simulink model "three_phase_inverter"  (R2025a)
settings: Solver=VariableStepAuto  StartTime=0.0  StopTime=1  FixedStep=step_time
undefined symbols (not defined in the file): fsw, Ls, Rs, Vdc
libraries: spsMosfetLib x6, spsVoltageMeasurementLib x6, spsCurrentMeasurementLib x3, spsDCVoltageSourceLib x2, ee_lib x2, nesl_utility x1, spsThreePhaseSeriesRLCBranchLib x1, fl_lib x1, spspowerguiLib x1
settings Model: Creator=moon  LastModifiedBy=moon

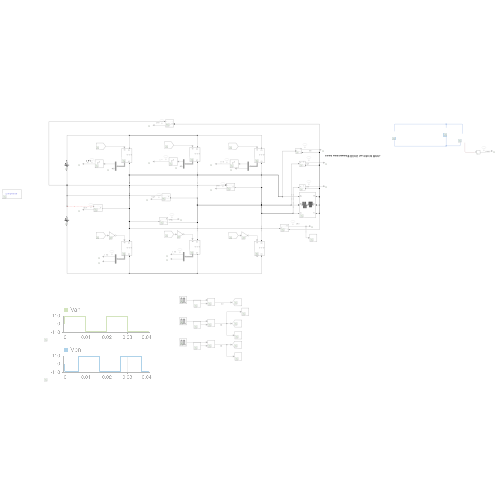
[thumbnail: Simulink's stored preview of the top-level diagram]
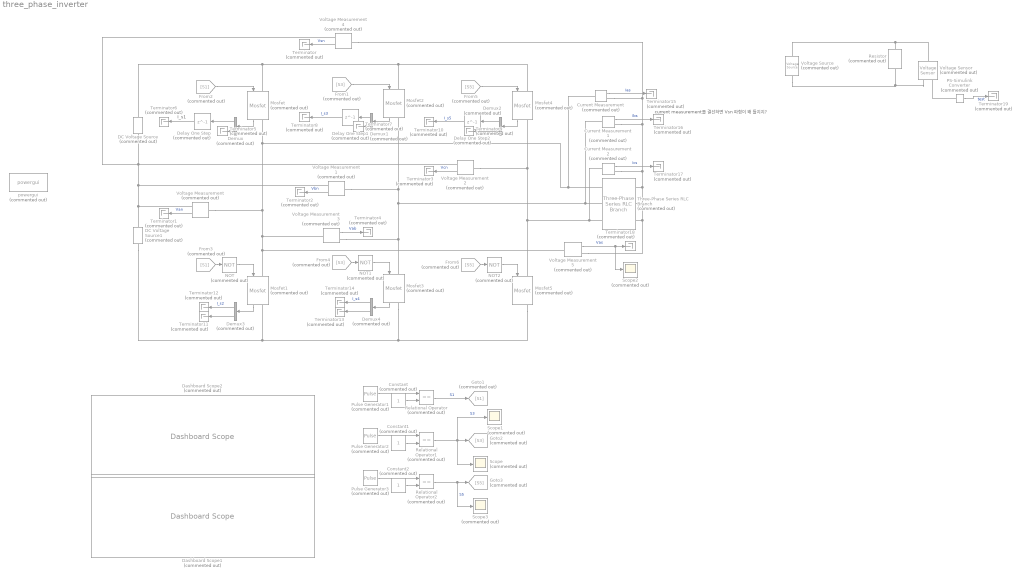
== system three_phase_inverter ==
  note: I_s1
  note: current measurement를 결선하면 Vsn 파형이 왜 틀지지?
  Constant : Constant  Commented=on
  Constant1 : Constant  Commented=on
  Constant2 : Constant  Commented=on
  Current Measurement : spsCurrentMeasurementLib/Current Measurement  Commented=on  PhasorSimulation=off  OutputType=Complex  PSBequivalent=0
  Current Measurement1 : spsCurrentMeasurementLib/Current Measurement  Commented=on  PhasorSimulation=off  OutputType=Complex  PSBequivalent=0
  Current Measurement2 : spsCurrentMeasurementLib/Current Measurement  Commented=on  PhasorSimulation=off  OutputType=Complex  PSBequivalent=0
  DC Voltage Source : spsDCVoltageSourceLib/DC Voltage Source  Commented=on  Amplitude=Vdc  Measurements=None
  DC Voltage Source1 : spsDCVoltageSourceLib/DC Voltage Source  Commented=on  Amplitude=Vdc  Measurements=None
  Dashboard Scope1 : DashboardScope  Commented=on  FontColor=[0.0, 0.0, 0.0]
  Dashboard Scope2 : DashboardScope  Commented=on  FontColor=[0.0, 0.0, 0.0]
  Delay One Step : Delay  Commented=on  DelayLength=1
  Delay One Step1 : Delay  Commented=on  DelayLength=1
  Delay One Step2 : Delay  Commented=on  DelayLength=1
  Demux{,1..4} (5 alike) : Demux  Commented=on  Outputs=2
  From1 : From  Commented=on  GotoTag=S3
  From2 : From  Commented=on  GotoTag=S1
  From3 : From  Commented=on  GotoTag=S1
  From4 : From  Commented=on  GotoTag=S3
  From5 : From  Commented=on  GotoTag=S5
  From6 : From  Commented=on  GotoTag=S5
  Goto1 : Goto  Commented=on  GotoTag=S1
  Goto2 : Goto  Commented=on  GotoTag=S3
  Goto3 : Goto  Commented=on  GotoTag=S5
  Mosfet{,1..5} (6 alike) : spsMosfetLib/Mosfet  Commented=on  Ron=R_FET  Lon=0  Rd=R_Diode  Vfd=0  IC=0  Rs=1e5  Cs=inf  Measurements=on
  NOT : Logic  Commented=on  Operator=NOT  IconShape=distinctive  AllPortsSameDT=off  OutDataTypeStr=boolean
  NOT1 : Logic  Commented=on  Operator=NOT  IconShape=distinctive  AllPortsSameDT=off  OutDataTypeStr=boolean
  NOT2 : Logic  Commented=on  Operator=NOT  IconShape=distinctive  AllPortsSameDT=off  OutDataTypeStr=boolean
  PS-Simulink Converter : nesl_utility/PS-Simulink Converter  Commented=on  PhysicalDomain=network_engine_domain  SubClassName=ps_output  LeftPortType=input  RightPortType=output  PseudoPeriodic=off  Frequencies=[]  VectorFormat=inherit  Unit=inherit  AffineConversion=off
  Pulse Generator1 : DiscretePulseGenerator  Commented=on  PulseType=Time based  Period=1/fsw  PulseWidth=50
  Pulse Generator2 : DiscretePulseGenerator  Commented=on  PulseType=Time based  Period=1/fsw  PulseWidth=50  PhaseDelay=1/fsw/3
  Pulse Generator3 : DiscretePulseGenerator  Commented=on  PulseType=Time based  Period=1/fsw  PulseWidth=50  PhaseDelay=-1/fsw/3
  Relational Operator : RelationalOperator  Commented=on  Operator===  OutDataTypeStr=boolean  RndMeth=Simplest  InputSameDT=off
  Relational Operator1 : RelationalOperator  Commented=on  Operator===  OutDataTypeStr=boolean  RndMeth=Simplest  InputSameDT=off
  Relational Operator2 : RelationalOperator  Commented=on  Operator===  OutDataTypeStr=boolean  RndMeth=Simplest  InputSameDT=off
  Resistor : ee_lib/Passive/Resistor  Commented=on  R=1 Ohm  enable_R_tol=ee.enum.toleranceApplication.none  R_tol=5  tol_distribution=ee.enum.toleranceDistribution.uniform  nSigma=4  enable_operating_limits=ee.enum.enable.no  operating_limit_action=ee.enum.passive.reportOpLim.warn  power_rating=1 W  max_working_voltage=100 V  noise_mode=ee.enum.sources.noise.Disabled  Tdevice=25 degC  sample_time=1e-3 s  repeatability=ee.enum.ic.repeatability.notRepeatable  user_seed=0  auto_seed=2715962282  power_derating_T1=70 degC  power_derating_T2=155 degC  operating_temperature_range_vec=[-50, 150] degC  alpha=3.93e-3 1/K  Tmeas=25 degC  thermal_mass=100 J/K  temperature_specify=off  temperature_priority=High  temperature=298.15 K  temperature_nominal_specify=off  temperature_nominal_value=1  temperature_nominal_unit=K
  Scope{,1..3} (4 alike) : Scope  Commented=on
      Scope settings: ActiveDisplayYMinimum=-0.12499999999999997  ActiveDisplayYMaximum=1.125
      Scope1 settings: ActiveDisplayYMinimum=-0.12499999999999997  ActiveDisplayYMaximum=1.125
      Scope2 settings: ActiveDisplayYMinimum=-166.66666666666666  ActiveDisplayYMaximum=166.66666666666663  DataLoggingVariableName=ScopeData2
      Scope3 settings: ActiveDisplayYMinimum=-1  ActiveDisplayYMaximum=1  DataLoggingVariableName=ScopeData3
  Terminator{,1..19} (20 alike) : Terminator  Commented=on
  Three-Phase Series RLC Branch : spsThreePhaseSeriesRLCBranchLib/Three-Phase Series RLC Branch  Commented=on  LConnTagsString=A|B|C  RConnTagsString=A|B|C  BranchType=RL  Resistance=Rs  Inductance=Ls  Capacitance=1e-6  Measurements=Branch voltages and currents
  Voltage Measurement : spsVoltageMeasurementLib/Voltage Measurement  Commented=on  PhasorSimulation=off  OutputType=Complex  PSBequivalent=0
      link override -: Side=Right
  Voltage Measurement1 : spsVoltageMeasurementLib/Voltage Measurement  Commented=on  PhasorSimulation=off  OutputType=Complex  PSBequivalent=0
      link override -: Side=Right
  Voltage Measurement2 : spsVoltageMeasurementLib/Voltage Measurement  Commented=on  PhasorSimulation=off  OutputType=Complex  PSBequivalent=0
      link override -: Side=Right
  Voltage Measurement3 : spsVoltageMeasurementLib/Voltage Measurement  Commented=on  PhasorSimulation=off  OutputType=Complex  PSBequivalent=0
      link override -: Side=Right
  Voltage Measurement4 : spsVoltageMeasurementLib/Voltage Measurement  Commented=on  PhasorSimulation=off  OutputType=Complex  PSBequivalent=0
      link override -: Side=Right
  Voltage Measurement5 : spsVoltageMeasurementLib/Voltage Measurement  Commented=on  PhasorSimulation=off  OutputType=Complex  PSBequivalent=0
      link override -: Side=Right
  Voltage Sensor : fl_lib/Electrical/Electrical Sensors/Voltage Sensor  Commented=on
  Voltage Source : ee_lib/Sources/Voltage Source  Commented=on  dc_voltage=0 V  ac_voltage=0 V  ac_shift=0 rad  ac_frequency=60 Hz  noise_mode=ee.enum.sources.noise.Disabled  PSD=0 V^2/Hz  sample_time=1e-3 s  repeatability=ee.enum.sources.repeatability.NotRepeatable  user_seed=0  auto_seed=545404223  i_specify=off  i_priority=None  i=0 A  i_nominal_specify=off  i_nominal_value=1  i_nominal_unit=A  v_specify=off  v_priority=None  v=0 V  v_nominal_specify=off  v_nominal_value=1  v_nominal_unit=V
  powergui : spspowerguiLib/powergui  Priority=1  Commented=on  SimulationMode=Continuous  SampleTime=50e-6  frequency=60  Iterations=50  frequencyindice=0  Pbase=100e6  ErrMax=1e-4  UnitsV=kV  UnitsW=MW  buscounter=0  FunctionMessages=off  echomessages=off  EnableUseOfTLC=off  CurrentSourceSwitches=off  DisableSnubberDevices=off  DisableRonSwitches=off  DisableVfSwitches=off  DisplayEquations=off  AutomaticDiscreteSolvers=off  SolverType=Tustin/Backward Euler (TBE)  Interpol=off  ExternalGateDelay=off  methode=off  Ts=100  x0status=blocks  SPID=on  SwTol=0  HookPort=off  NonlinearTolerance=1e-4  nMaxIteration=100  ContinueOnMaxIteration=off  RestoreLinks=warning  ResistiveCurrentMeasurement=off  Frange=[0:2:500]  Ylog=off  Xlog=on  ShowGrid=off  save=off  variable=ZData  structure=0  ZoomFFT=off  StartTime=0.0  cycles=1  DisplayStyle=1  fundamental=60  FreqAxis=off  MaxFrequency=1000  frequencyindicesteady=1  RmsSteady=1  display=off
  wires:
  Voltage Measurement/1 -> Terminator1/1  "Van"
  From2/1 -> Mosfet/1
  Pulse Generator1/1 -> Relational Operator/1
  Constant/1 -> Relational Operator/2
  Relational Operator/1 -> Goto1/1  "S1"
  From3/1 -> NOT/1
  NOT/1 -> Mosfet1/1
  Relational Operator1/1 -> Scope/1, Scope1/1, Goto2/1  "S3"
  Pulse Generator2/1 -> Relational Operator1/1
  Constant1/1 -> Relational Operator1/2
  Relational Operator2/1 -> Scope3/1, Goto3/1  "S5"
  Constant2/1 -> Relational Operator2/2
  Pulse Generator3/1 -> Relational Operator2/1
  From4/1 -> NOT1/1
  Voltage Measurement1/1 -> Terminator2/1  "Vbn"
  NOT1/1 -> Mosfet3/1
  From1/1 -> Mosfet2/1
  From6/1 -> NOT2/1
  Voltage Measurement2/1 -> Terminator3/1  "Vcn"
  NOT2/1 -> Mosfet5/1
  From5/1 -> Mosfet4/1
  Voltage Measurement3/1 -> Terminator4/1  "Vab"
  Voltage Measurement4/1 -> Terminator/1  "Vsn"
  Current Measurement/1 -> Terminator15/1  "Ias"
  Mosfet/1 -> Demux/1
  Demux/2 -> Terminator5/1
  Demux1/2 -> Terminator7/1
  Delay One Step1/1 -> Terminator8/1  "I_s3"
  Mosfet2/1 -> Demux1/1
  Demux2/2 -> Terminator9/1
  Demux2/1 -> Delay One Step2/1
  Mosfet4/1 -> Demux2/1
  Demux3/2 -> Terminator11/1
  Demux3/1 -> Terminator12/1  "I_s2"
  Mosfet1/1 -> Demux3/1
  Demux4/2 -> Terminator13/1
  Mosfet3/1 -> Demux4/1
  Demux4/1 -> Terminator14/1  "I_s4"
  Current Measurement1/1 -> Terminator16/1  "Ibs"
  Current Measurement2/1 -> Terminator17/1  "Ics"
  Demux/1 -> Delay One Step/1
  Delay One Step/1 -> Terminator6/1
  Demux1/1 -> Delay One Step1/1
  Delay One Step2/1 -> Terminator10/1  "I_s5"
  Voltage Measurement5/1 -> Scope2/1, Terminator18/1  "Vas"
  PS-Simulink Converter/1 -> Terminator19/1  "test"
  connections:
  DC Voltage Source1/RConn1 -- Voltage Measurement/RConn1 -- Voltage Measurement2/RConn1 -- Voltage Measurement4/RConn1 -- DC Voltage Source/LConn1 -- Voltage Measurement1/RConn1
  DC Voltage Source/RConn1 -- Mosfet4/LConn1 -- Mosfet2/LConn1 -- Mosfet/LConn1
  Mosfet1/LConn1 -- Voltage Measurement/LConn1 -- Three-Phase Series RLC Branch/LConn1 -- Current Measurement/LConn1 -- Mosfet/RConn1 -- Voltage Measurement3/LConn1 -- Voltage Measurement5/LConn1
  DC Voltage Source1/LConn1 -- Mosfet1/RConn1 -- Mosfet3/RConn1 -- Mosfet5/RConn1
  Mosfet3/LConn1 -- Voltage Measurement3/RConn1 -- Current Measurement1/LConn1 -- Three-Phase Series RLC Branch/LConn2 -- Voltage Measurement1/LConn1 -- Mosfet2/RConn1
  Mosfet5/LConn1 -- Current Measurement2/LConn1 -- Three-Phase Series RLC Branch/LConn3 -- Voltage Measurement2/LConn1 -- Mosfet4/RConn1
  Three-Phase Series RLC Branch/RConn3 -- Three-Phase Series RLC Branch/RConn2 -- Current Measurement1/RConn1 -- Voltage Measurement4/LConn1 -- Current Measurement/RConn1 -- Current Measurement2/RConn1 -- Three-Phase Series RLC Branch/RConn1 -- Voltage Measurement5/RConn1
  Voltage Source/LConn1 -- Voltage Sensor/LConn1 -- Resistor/LConn1
  Voltage Source/RConn1 -- Voltage Sensor/RConn2 -- Resistor/RConn1
  PS-Simulink Converter/LConn1 -- Voltage Sensor/RConn1
